simulink model "modelSFDcrte"  (R2021a)
settings: Solver=VariableStepAuto  StartTime=0.0  StopTime=10.0  RelTol=1e-3
values from neighbouring files (symbols this model uses):
  Gd = c2d(G,Ts,'zoh')    [BuildGridCustom.m]    (also in uMPC.m)
  Ts = 0.01    [BuildGridCustom.m]    (also in workspacesetup.m = 0.02)
  Weh = c2d(We,Ts,'Tustin')    [BuildGridCustom.m]
  Wev = c2d(We,Ts,'Tustin')    [BuildGridCustom.m]
  Wuh = c2d(Wu,Ts,'Tustin')    [BuildGridCustom.m]
  Wuv = c2d(Wu,Ts,'Tustin')    [BuildGridCustom.m]
settings Model: Creator=ariel  LastModifiedBy=ariel

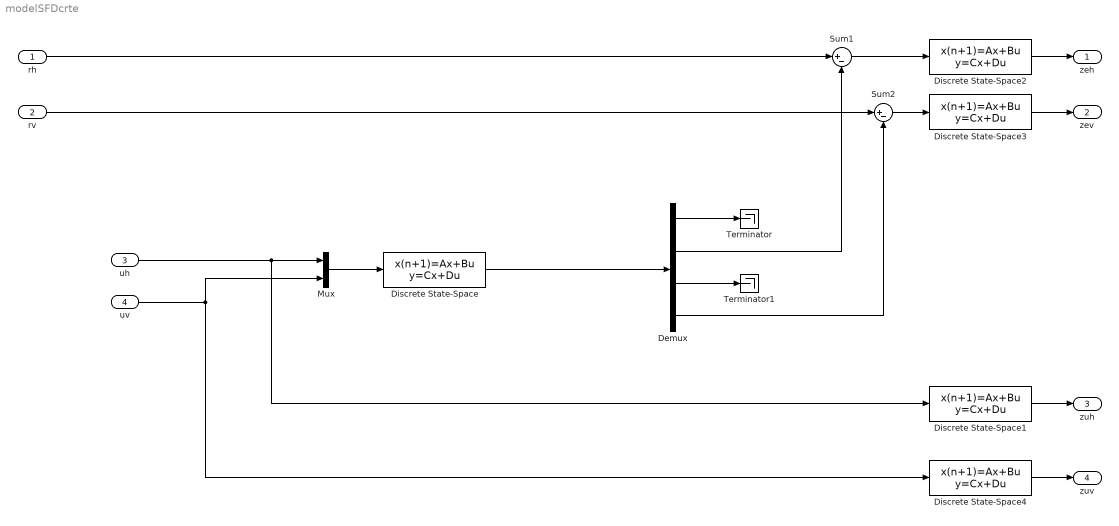
== system modelSFDcrte ==
  rh : Inport  PortDimensions=1
  rv : Inport  Port=2  PortDimensions=1
  uh : Inport  Port=3  PortDimensions=1
  uv : Inport  Port=4  PortDimensions=1
  Demux : Demux
  Discrete State-Space : DiscreteStateSpace  A=Gd.A  B=Gd.B  C=Gd.C  D=Gd.D  SampleTime=Ts
  Discrete State-Space1 : DiscreteStateSpace  A=Wuh.A  B=Wuh.B  C=Wuh.C  D=Wuh.D  SampleTime=Ts
  Discrete State-Space2 : DiscreteStateSpace  A=Weh.A  B=Weh.B  C=Weh.C  D=Weh.D  SampleTime=Ts
  Discrete State-Space3 : DiscreteStateSpace  A=Wev.A  B=Wev.B  C=Wev.C  D=Wev.D  SampleTime=Ts
  Discrete State-Space4 : DiscreteStateSpace  A=Wuv.A  B=Wuv.B  C=Wuv.C  D=Wuv.D  SampleTime=Ts
  Mux : Mux  Inputs=2
  Sum1 : Sum  Inputs=|+-
  Sum2 : Sum  Inputs=|+-
  Terminator : Terminator
  Terminator1 : Terminator
  zeh : Outport  PortDimensions=1
  zev : Outport  Port=2  PortDimensions=1
  zuh : Outport  Port=3  PortDimensions=1
  zuv : Outport  Port=4  PortDimensions=1
  wires:
  Discrete State-Space/1 -> Demux/1
  rh/1 -> Sum1/1
  uh/1 -> Discrete State-Space1/1, Mux/1
  Discrete State-Space1/1 -> zuh/1
  Sum1/1 -> Discrete State-Space2/1
  Discrete State-Space2/1 -> zeh/1
  Demux/2 -> Sum1/2
  Demux/1 -> Terminator/1
  Demux/3 -> Terminator1/1
  Sum2/1 -> Discrete State-Space3/1
  Discrete State-Space3/1 -> zev/1
  Demux/4 -> Sum2/2
  rv/1 -> Sum2/1
  Discrete State-Space4/1 -> zuv/1
  uv/1 -> Discrete State-Space4/1, Mux/2
  Mux/1 -> Discrete State-Space/1
